simulink model "UNIPG_Modell"  (R2021a)
settings: Solver=ode1  StartTime=0.0  StopTime=t_Stop  FixedStep=0.1  RelTol=1e-3
values from neighbouring files (symbols this model uses):
  b = 0.7    [ParameterBarccesiUNIPG.m]
  k = 1.414    [ParameterBarccesiUNIPG.m]
  k_x = 0.84    [ParameterBarccesiUNIPG.m]
  k_y = 3.36    [ParameterBarccesiUNIPG.m]
  k_z = 0.84    [ParameterBarccesiUNIPG.m]
  mue = 900    [ParameterBarccesiUNIPG.m]
  n = 2    [ParameterBarccesiUNIPG.m]
  P = 0.85    [ParameterBarccesiUNIPG.m]
  tau_x = 0.6    [ParameterBarccesiUNIPG.m]
  tau_y = 2.4    [ParameterBarccesiUNIPG.m]
  tau_z = 0.6    [ParameterBarccesiUNIPG.m]
settings Model: Creator=BattiPerdator  LastModifiedBy=BattiPerdator
settings DebuggingCC: SignalInfNanChecking=error

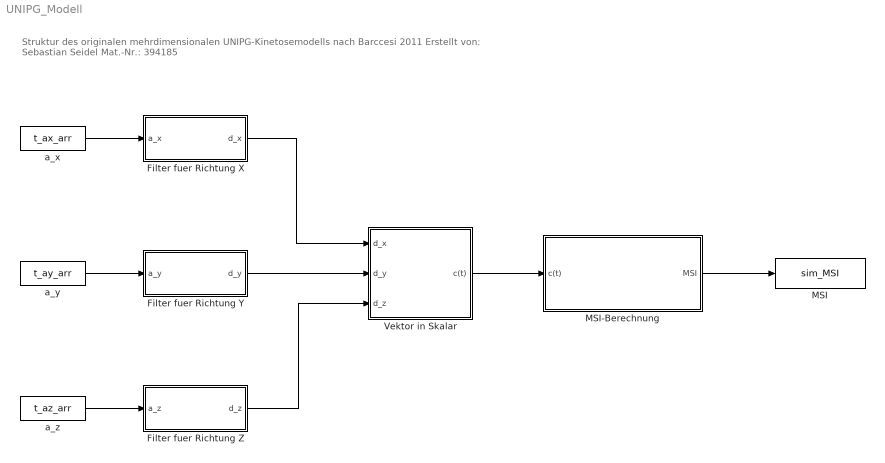
== system UNIPG_Modell ==
  note: Struktur des originalen mehrdimensionalen UNIPG-Kinetosemodells nach Barccesi 2011
      | Erstellt von: Sebastian Seidel
      | Mat.-Nr.: 394185
  Filter fuer Richtung X : Subsystem
  Filter fuer Richtung Y : Subsystem
  Filter fuer Richtung Z : Subsystem
  MSI : ToWorkspace  VariableName=sim_MSI  SampleTime=-1
  MSI-Berechnung : Subsystem
  Vektor in Skalar : Subsystem
  a_x : FromWorkspace  VariableName=t_ax_arr
  a_y : FromWorkspace  VariableName=t_ay_arr
  a_z : FromWorkspace  VariableName=t_az_arr
  wires:
  a_x/1 -> Filter fuer Richtung X/1(a_x)
  a_y/1 -> Filter fuer Richtung Y/1(a_y)
  a_z/1 -> Filter fuer Richtung Z/1(a_z)
  Filter fuer Richtung X/1(d_x) -> Vektor in Skalar/1(d_x)
  Filter fuer Richtung Y/1(d_y) -> Vektor in Skalar/2(d_y)
  Filter fuer Richtung Z/1(d_z) -> Vektor in Skalar/3(d_z)
  Vektor in Skalar/1(c(t)) -> MSI-Berechnung/1(c(t))
  MSI-Berechnung/1(MSI) -> MSI/1

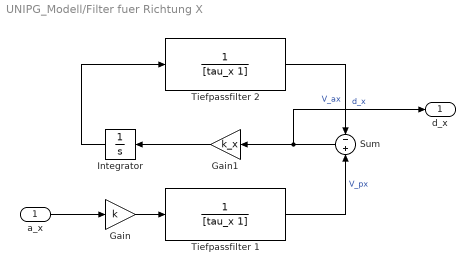
== system UNIPG_Modell/Filter fuer Richtung X ==
  a_x : Inport
  Gain : Gain  Gain=k
  Gain1 : Gain  Gain=k_x
  Integrator : Integrator
  Sum : Sum  Inputs=-|+
  Tiefpassfilter 1 : TransferFcn  Denominator=[tau_x 1]
  Tiefpassfilter 2 : TransferFcn  Denominator=[tau_x 1]
  d_x : Outport
  wires:
  a_x/1 -> Gain/1
  Gain/1 -> Tiefpassfilter 1/1
  Tiefpassfilter 1/1 -> Sum/2  "V_px"
  Sum/1 -> d_x/1, Gain1/1  "d_x"
  Gain1/1 -> Integrator/1
  Integrator/1 -> Tiefpassfilter 2/1
  Tiefpassfilter 2/1 -> Sum/1  "V_ax"

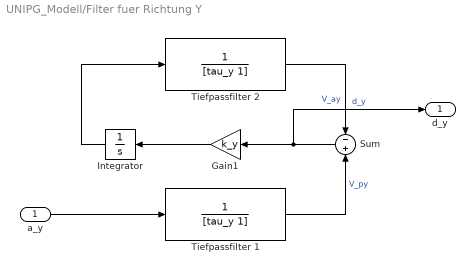
== system UNIPG_Modell/Filter fuer Richtung Y ==
  a_y : Inport
  Gain1 : Gain  Gain=k_y
  Integrator : Integrator
  Sum : Sum  Inputs=-|+
  Tiefpassfilter 1 : TransferFcn  Denominator=[tau_y 1]
  Tiefpassfilter 2 : TransferFcn  Denominator=[tau_y 1]
  d_y : Outport
  wires:
  Sum/1 -> d_y/1, Gain1/1  "d_y"
  Tiefpassfilter 1/1 -> Sum/2  "V_py"
  Gain1/1 -> Integrator/1
  Integrator/1 -> Tiefpassfilter 2/1
  Tiefpassfilter 2/1 -> Sum/1  "V_ay"
  a_y/1 -> Tiefpassfilter 1/1

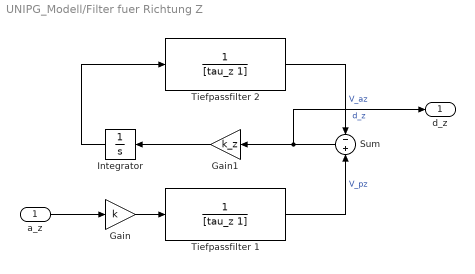
== system UNIPG_Modell/Filter fuer Richtung Z ==
  a_z : Inport
  Gain : Gain  Gain=k
  Gain1 : Gain  Gain=k_z
  Integrator : Integrator
  Sum : Sum  Inputs=-|+
  Tiefpassfilter 1 : TransferFcn  Denominator=[tau_z 1]
  Tiefpassfilter 2 : TransferFcn  Denominator=[tau_z 1]
  d_z : Outport
  wires:
  Integrator/1 -> Tiefpassfilter 2/1
  Tiefpassfilter 2/1 -> Sum/1  "V_az"
  Gain1/1 -> Integrator/1
  Gain/1 -> Tiefpassfilter 1/1
  a_z/1 -> Gain/1
  Tiefpassfilter 1/1 -> Sum/2  "V_pz"
  Sum/1 -> d_z/1, Gain1/1  "d_z"

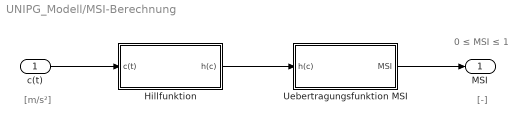
== system UNIPG_Modell/MSI-Berechnung ==
  note: 0 ≤ MSI ≤ 1
  note: [-]
  note: [m/s²]
  c(t) : Inport
  Hillfunktion : Subsystem
  Uebertragungsfunktion MSI : Subsystem
  MSI : Outport
  wires:
  c(t)/1 -> Hillfunktion/1(c(t))
  Uebertragungsfunktion MSI/1(MSI) -> MSI/1
  Hillfunktion/1(h(c)) -> Uebertragungsfunktion MSI/1(h(c))

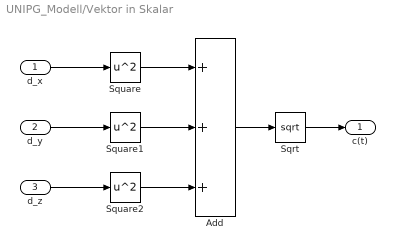
== system UNIPG_Modell/Vektor in Skalar ==
  d_x : Inport
  d_y : Inport  Port=2
  d_z : Inport  Port=3
  Add : Sum  Inputs=+++
  Sqrt : Sqrt  SaturateOnIntegerOverflow=on
  Square : Math  Operator=square  SaturateOnIntegerOverflow=on
  Square1 : Math  Operator=square  SaturateOnIntegerOverflow=on
  Square2 : Math  Operator=square  SaturateOnIntegerOverflow=on
  c(t) : Outport
  wires:
  Add/1 -> Sqrt/1
  Square2/1 -> Add/3
  Square1/1 -> Add/2
  Square/1 -> Add/1
  d_x/1 -> Square/1
  d_y/1 -> Square1/1
  d_z/1 -> Square2/1
  Sqrt/1 -> c(t)/1

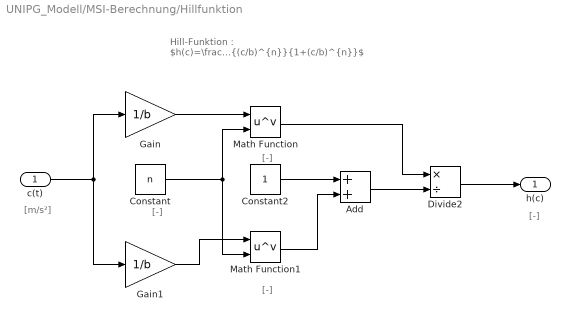
== system UNIPG_Modell/MSI-Berechnung/Hillfunktion ==
  note: Hill-Funktion :
      | $h(c)=\frac{(c/b)^{n}}{1+(c/b)^{n}}$
  note: [-]
  note: [-]
  note: [-]
  note: [m/s²]
  note: [-]
  c(t) : Inport
  Add : Sum
  Constant : Constant  Value=n
  Constant2 : Constant
  Divide2 : Product  Inputs=*/
  Gain : Gain  Gain=1/b
  Gain1 : Gain  Gain=1/b
  Math Function : Math  Operator=pow  SaturateOnIntegerOverflow=on
  Math Function1 : Math  Operator=pow  SaturateOnIntegerOverflow=on
  h(c) : Outport
  wires:
  Constant2/1 -> Add/1
  Math Function1/1 -> Add/2
  Divide2/1 -> h(c)/1
  Add/1 -> Divide2/2
  Math Function/1 -> Divide2/1
  Constant/1 -> Math Function1/2, Math Function/2
  Gain/1 -> Math Function/1
  Gain1/1 -> Math Function1/1
  c(t)/1 -> Gain1/1, Gain/1

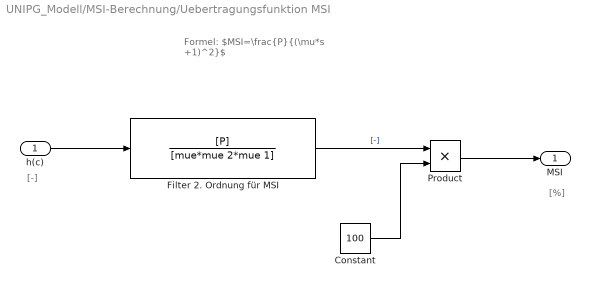
== system UNIPG_Modell/MSI-Berechnung/Uebertragungsfunktion MSI ==
  note: Formel:
      | $MSI=\frac{P}{(\mu*s +1)^2}$
  note: [%]
  note: [-]
  h(c) : Inport
  Constant : Constant  Value=100
  Filter 2. Ordnung für MSI : TransferFcn  Numerator=[P]  Denominator=[mue*mue 2*mue 1]  ParameterTunability=Optimized
  Product : Product
  MSI : Outport
  wires:
  h(c)/1 -> Filter 2. Ordnung für MSI/1
  Product/1 -> MSI/1
  Filter 2. Ordnung für MSI/1 -> Product/1  "[-]"
  Constant/1 -> Product/2
